simulink model "OOK_2400_2020b"  (R2020b)
settings: Solver=VariableStepDiscrete  StartTime=0.0  StopTime=4000/Rb  RelTol=1e-3  EnableMultiTasking=on
PreLoadFcn:
  | fc=30000;
  | Rb=2400;
libraries: commrandsrc2 x1
settings Model: Creator=morelos_zaragoza  LastModifiedBy=14083
settings DataIOCC: LimitDataPoints=on  SaveFormat=Array  SignalLoggingSaveFormat=ModelDataLogs  ReturnWorkspaceOutputs=off
settings OptimizationCC: ExpressionDepthLimit=2147483647  InitFltsAndDblsToZero=on  LifeSpan=inf
settings DebuggingCC: SaveWithParameterizedLinksMsg=none  UnderspecifiedInitializationDetection=Classic  MergeDetectMultiDrivingBlocksExec=none  SignalResolutionControl=TryResolveAllWithWarning  SolverPrmCheckMsg=warning  MultiTaskDSMMsg=warning  MultiTaskCondExecSysMsg=none  FcnCallInpInsideContextMsg=warning  StateNameClashWarn=warning  SFUnexpectedBacktrackingDiag=warning  SFNoUnconditionalDefaultTransitionDiag=warning  SFExecutionAtInitializationDiag=none  ArithmeticOperatorsInVariantConditions=warning
settings HardwareCC: ProdBitPerPointer=32  ProdBitPerSizeT=32  ProdBitPerPtrDiffT=32  ProdLargestAtomicFloat=None  ProdIntDivRoundTo=Undefined  ProdEndianess=Unspecified  ProdWordSize=32  ProdHWDeviceType=32-bit Generic
settings ModelReferenceCC: PropagateSignalLabelsOutOfModel=off
settings SFSimCC: SimUseLocalCustomCode=off  CustomCodeUndefinedFunction=UseInterfaceOnly
settings RTWCC: RTWUseLocalCustomCode=off
settings CodeAppCC: StateflowObjectComments=on
settings GRTTargetCC: TargetFcnLib=ansi_tfl_tmw.mat  TargetLangStandard=C89/C90 (ANSI)  CombineOutputUpdateFcns=off  GRTInterface=on
settings ConfigComp: CovMetricSettings=dw  CovSaveCumulativeToWorkspaceVar=on  CovSaveSingleToWorkspaceVar=on  CovExternalEMLEnable=off

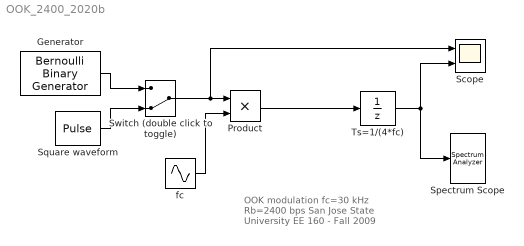
== system OOK_2400_2020b ==
  note: OOK modulation
      | fc=30 kHz
      | Rb=2400 bps
      | San Jose State University
      | EE 160 - Fall 2009
  Generator : commrandsrc2/Bernoulli Binary Generator  P=1/2  seed=37511  Ts=1/Rb  frameBased=off  sampPerFrame=1  orient=off  outDataType=double
      settings: SourceProductBaseCode=CM
  Product : Product  RndMeth=Zero
  Scope : Scope  NumInputPorts=2
  Spectrum Scope : SpectrumAnalyzer
  Square waveform : DiscretePulseGenerator  PulseType=Time based  Period=2/Rb  PulseWidth=50
  Switch (double click to toggle) : ManualSwitch  CurrentSetting=0
  Ts=1/(4*fc) : UnitDelay  SampleTime=1/(4*fc)  HasFrameUpgradeWarning=on
  fc : Sin  Frequency=2*pi*fc  SampleTime=1/(16*fc)
  wires:
  Switch (double click to toggle)/1 -> Product/1, Scope/1
  fc/1 -> Product/2
  Ts=1/(4*fc)/1 -> Scope/2, Spectrum Scope/1
  Product/1 -> Ts=1/(4*fc)/1
  Generator/1 -> Switch (double click to toggle)/1
  Square waveform/1 -> Switch (double click to toggle)/2
